simulink model "ee463_term_project"  (R2020a)
settings: Solver=VariableStepAuto  StartTime=0.0  StopTime=20  RelTol=1e-3
undefined symbols (not defined in the file): Acid, Lead
libraries: powerlib x25, electricdrivelib x1, powerlib_meascontrol x1, eePwmGenerator x1
settings Model: Creator=görkem  LastModifiedBy=görkem

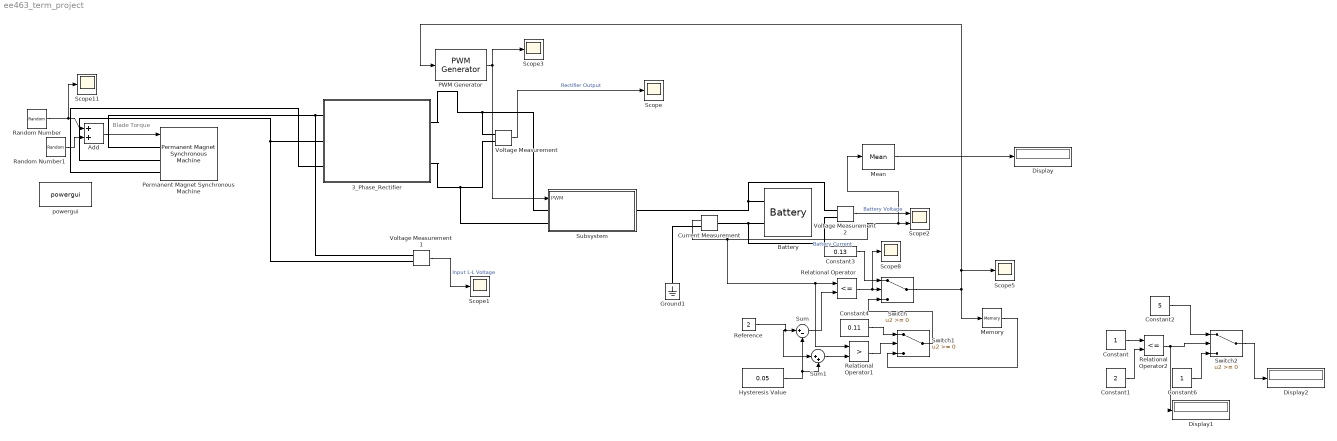
== system ee463_term_project ==
  note: Blade Torque
  3_Phase_Rectifier : Subsystem
  Add : Sum
  Battery : electricdrivelib/Extra Sources/Battery  BatType=Lead-Acid  ShowTempParam=off  ThermalPreset=no  ShowAgeParam=off  NomV=24  NomQ=5.4  SOC=50  Batt_Tr=30  PresetModel=on  MaxQ=5.625  MinV=18  FullV=26.1316  Dis_rate=1.08  R=0.044444  Normal_OP=1.6755  expZone="[24.4342        0.018]"  current=[6.5 13 32.5]  Units=Time  Tci=20  NomT=20  T2=-30  MaxQ2=4.8  FullV2=7.1  Normal_OP2=5.655  expZone2="[6.58           1]"  Rca=0.6  ti=2000  Dp=0  Neq0=0  Tsim=1e6  Ta1=25  Qeol=5.4*0.9  Reol=0.013333*1.2  Char_age=[2.3478, 3]  Dis_age=[2.3478, 10]  N1=1500  N2=10500  N3=1000  N4=1400  Ta2=45  N5=950
  Constant : Constant
  Constant1 : Constant  Value=2
  Constant2 : Constant  Value=5
  Constant3 : Constant  Value=0.13
  Constant4 : Constant  Value=0.11
  Constant6 : Constant
  Current Measurement : powerlib/Measurements/Current Measurement  PhasorSimulation=off  OutputType=Complex  PSBequivalent=0
  Display : Display
  Display1 : Display
  Display2 : Display
  Ground1 : powerlib/Elements/Ground  LConnTagsString=a
  Hysteresis Value : Constant  Value=0.05
  Mean : powerlib_meascontrol/Measurements/Mean  Freq=60  Vinit=0  Ts=0
  Memory : Memory
  PWM Generator : eePwmGenerator/PWM Generator  CarrCount=Up  Tper=0.0001  Ts=1e-5
  Permanent Magnet Synchronous Machine : powerlib/Machines/Permanent Magnet Synchronous Machine  NbPhases=3  FluxDistribution=Sinusoidal  RotorType=Round  MechanicalLoad=Torque Tm  PresetModel=No  ShowDetailedParameters=on  MeasurementBus=off  Resistance=10.58  Inductance=8.5e-3  dqInductances=[8.5e-3,8.5e-3]  La=0.0167  MachineConstant=Voltage Constant (V_peak L-L / krpm)  Flux=0.60646  VoltageCst=110  TorqueCst=0.90969  Flat=120  Mechanical=[0.00027 0.005024 1 0]  PolePairs=4  InitialConditions=[300,0, 0,0]  InitialConditions5ph=[0 0 0 0 0 0]  RefAngle=90 degrees behind phase A axis (modified Park)  IterativeDiscreteModel=Trapezoidal non iterative  TsBlock=-1  TsPowergui=0
  Random Number : RandomNumber  Mean=-1.6  Variance=0.05  SampleTime=1
  Random Number1 : RandomNumber  Variance=0.1  SampleTime=1e-3
  Reference : Constant  Value=2
  Relational Operator : RelationalOperator  Operator=<=  OutDataTypeStr=boolean  RndMeth=Simplest
  Relational Operator1 : RelationalOperator  Operator=>  OutDataTypeStr=boolean  RndMeth=Simplest
  Relational Operator2 : RelationalOperator  Operator=<=  OutDataTypeStr=boolean  RndMeth=Simplest
  Scope{,1,3,5,8,11} (6 alike) : Scope
  Scope2 : Scope  NumInputPorts=2
  Subsystem : Subsystem
  Sum : Sum  Inputs=|+-
  Sum1 : Sum  Inputs=|++
  Switch : Switch
  Switch1 : Switch
  Switch2 : Switch
  Voltage Measurement : powerlib/Measurements/Voltage Measurement  PhasorSimulation=off  OutputType=Complex  PSBequivalent=0
  Voltage Measurement1 : powerlib/Measurements/Voltage Measurement  PhasorSimulation=off  OutputType=Complex  PSBequivalent=0
  Voltage Measurement2 : powerlib/Measurements/Voltage Measurement  PhasorSimulation=off  OutputType=Complex  PSBequivalent=0
  powergui : powerlib/powergui  Priority=1  SimulationMode=Discrete  SampleTime=1e-5  frequency=60  Iterations=50  frequencyindice=0  Pbase=100e6  ErrMax=1e-4  UnitsV=kV  UnitsW=MW  buscounter=0  FunctionMessages=off  echomessages=off  EnableUseOfTLC=off  CurrentSourceSwitches=off  DisableSnubberDevices=off  DisableRonSwitches=off  DisableVfSwitches=off  DisplayEquations=off  AutomaticDiscreteSolvers=off  SolverType=Tustin/Backward Euler (TBE)  Interpol=off  ExternalGateDelay=off  methode=off  Ts=100  x0status=blocks  SPID=on  SwTol=0  HookPort=off  NonlinearTolerance=1e-4  nMaxIteration=100  ContinueOnMaxIteration=off  RestoreLinks=warning  ResistiveCurrentMeasurement=off  Frange=[0:2:500]  Ylog=off  Xlog=on  ShowGrid=off  save=off  variable=ZData  structure=0  ZoomFFT=off  StartTime=0.0  cycles=1  DisplayStyle=1  fundamental=60  FreqAxis=off  MaxFrequency=1000  frequencyindicesteady=1  RmsSteady=1  display=off
  wires:
  Voltage Measurement/1 -> Scope/1  "Rectifier Output"
  PWM Generator/1 -> Scope3/1, Subsystem/1(PWM)
  Random Number/1 -> Scope11/1, Add/1
  Add/1 -> Permanent Magnet Synchronous Machine/1
  Voltage Measurement1/1 -> Scope1/1  "Input L-L Voltage"
  Voltage Measurement2/1 -> Scope2/1  "Battery Voltage"
  Current Measurement/1 -> Relational Operator1/1, Relational Operator/1, Mean/1, Scope2/2  "Battery Current"
  Random Number1/1 -> Add/2
  Reference/1 -> Sum1/1, Sum/1
  Sum/1 -> Relational Operator/2
  Hysteresis Value/1 -> Sum/2, Sum1/2
  Sum1/1 -> Relational Operator1/2
  Constant3/1 -> Switch/1
  Relational Operator/1 -> Scope8/1, Switch/2
  Switch1/1 -> Switch/3
  Constant4/1 -> Switch1/1
  Relational Operator1/1 -> Switch1/2
  Memory/1 -> Switch1/3
  Mean/1 -> Display/1
  Constant/1 -> Relational Operator2/1
  Constant1/1 -> Relational Operator2/2
  Relational Operator2/1 -> Display1/1, Switch2/2
  Constant2/1 -> Switch2/1
  Constant6/1 -> Switch2/3
  Switch2/1 -> Display2/1
  Switch/1 -> PWM Generator/1, Scope5/1, Memory/1
  connections:
  Current Measurement/LConn1 -- Voltage Measurement2/LConn2 -- Battery/LConn2
  3_Phase_Rectifier/LConn1 -- Permanent Magnet Synchronous Machine/LConn1 -- Voltage Measurement1/LConn1
  3_Phase_Rectifier/RConn2 -- Voltage Measurement/LConn2 -- Subsystem/LConn2
  3_Phase_Rectifier/LConn2 -- Permanent Magnet Synchronous Machine/LConn2 -- Voltage Measurement1/LConn2
  Voltage Measurement/LConn1 -- 3_Phase_Rectifier/RConn1 -- Subsystem/LConn1
  Voltage Measurement2/LConn1 -- Subsystem/RConn1 -- Battery/LConn1
  Permanent Magnet Synchronous Machine/LConn3 -- 3_Phase_Rectifier/LConn3
  Ground1/LConn1 -- Current Measurement/RConn1

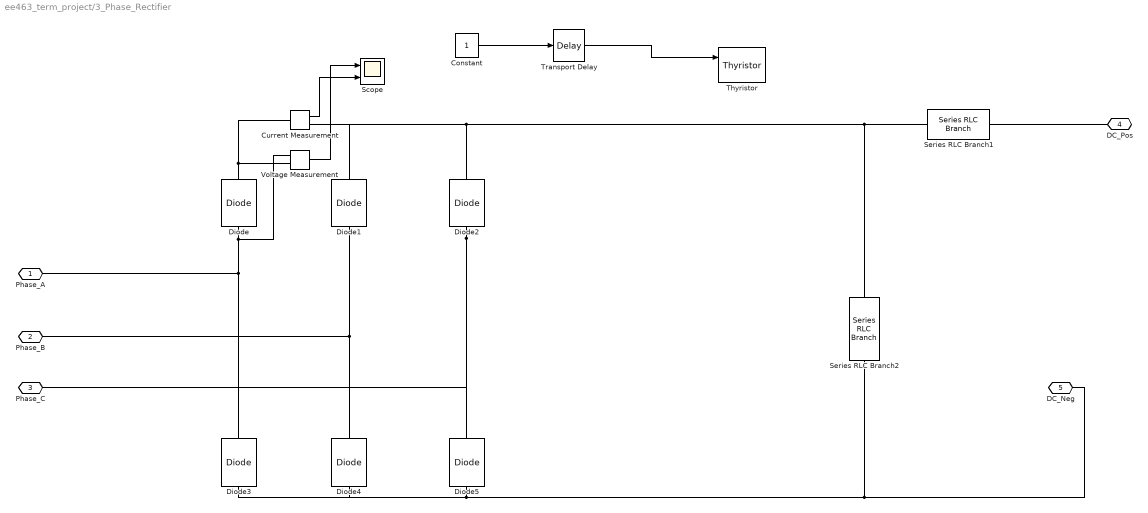
== system ee463_term_project/3_Phase_Rectifier ==
  Constant : Constant
  Current Measurement : powerlib/Measurements/Current Measurement  PhasorSimulation=off  OutputType=Complex  PSBequivalent=0
  Diode{,1..5} (6 alike) : powerlib/Power Electronics/Diode  Ron=0.001  Lon=0  Vf=0.8  IC=0  UseSnubber=0  Rs=500  Cs=250e-9  Measurements=off
  Scope : Scope  NumInputPorts=2
  Series RLC Branch1 : powerlib/Elements/Series RLC Branch  LConnTagsString=__new0  RConnTagsString=__new0  BranchType=R  Resistance=20  Inductance=1e-3  SetiL0=off  InitialCurrent=0  Capacitance=1e-6  Setx0=off  InitialVoltage=0  Measurements=None
  Series RLC Branch2 : powerlib/Elements/Series RLC Branch  LConnTagsString=__new0  RConnTagsString=__new0  BranchType=C  Resistance=72  Inductance=1e-3  SetiL0=off  InitialCurrent=0  Capacitance=1e-3  Setx0=off  InitialVoltage=0  Measurements=None
  Thyristor : powerlib/Power Electronics/Thyristor  Ron=0.001  Lon=0  Vf=0.8  IC=0  Rs=500  Cs=250e-9  Measurements=off
  Transport Delay : TransportDelay  DelayTime=0.2
  Voltage Measurement : powerlib/Measurements/Voltage Measurement  PhasorSimulation=off  OutputType=Complex  PSBequivalent=0
  Phase_A : PMIOPort  Side=Left
  Phase_B : PMIOPort  Port=2  Side=Left
  Phase_C : PMIOPort  Port=3  Side=Left
  DC_Pos : PMIOPort  Port=4  Side=Right
  DC_Neg : PMIOPort  Port=5  Side=Right
  wires:
  Transport Delay/1 -> Thyristor/1
  Constant/1 -> Transport Delay/1
  Voltage Measurement/1 -> Scope/1
  Current Measurement/1 -> Scope/2
  connections:
  Diode2/LConn1 -- Phase_C/RConn1 -- Diode5/RConn1
  Series RLC Branch2/LConn1 -- Current Measurement/RConn1 -- Diode1/RConn1 -- Diode2/RConn1 -- Series RLC Branch1/LConn1
  Series RLC Branch2/RConn1 -- Diode3/LConn1 -- Diode4/LConn1 -- Diode5/LConn1 -- DC_Neg/RConn1
  Phase_A/RConn1 -- Diode3/RConn1 -- Voltage Measurement/LConn1 -- Diode/LConn1
  Diode4/RConn1 -- Phase_B/RConn1 -- Diode1/LConn1
  Diode/RConn1 -- Current Measurement/LConn1 -- Voltage Measurement/LConn2
  Series RLC Branch1/RConn1 -- DC_Pos/RConn1

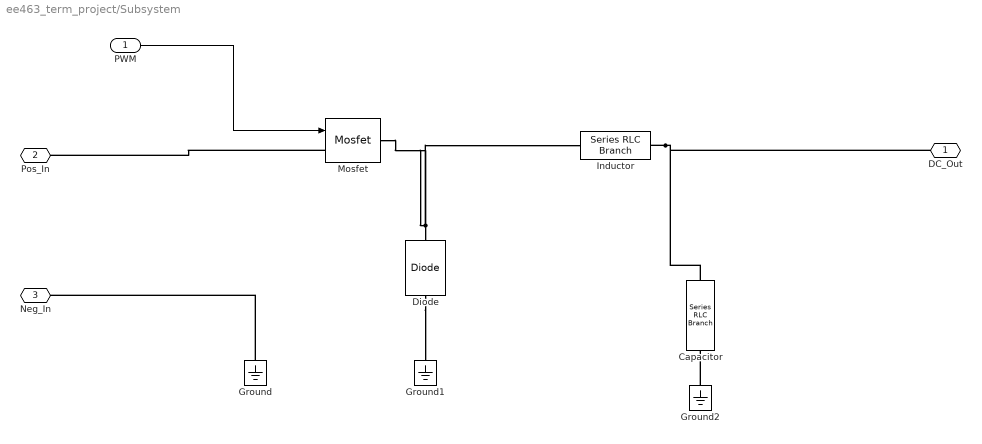
== system ee463_term_project/Subsystem ==
  PWM : Inport
  Capacitor : powerlib/Elements/Series RLC Branch  LConnTagsString=__new0  RConnTagsString=__new0  BranchType=C  Resistance=1  Inductance=1e-3  SetiL0=off  InitialCurrent=0  Capacitance=50e-6  Setx0=off  InitialVoltage=0  Measurements=None
  Diode : powerlib/Power Electronics/Diode  Ron=0.001  Lon=0  Vf=0.8  IC=0  UseSnubber=off  Rs=500  Cs=250e-9  Measurements=off
  Ground : powerlib/Elements/Ground  LConnTagsString=a
  Ground1 : powerlib/Elements/Ground  LConnTagsString=a
  Ground2 : powerlib/Elements/Ground  LConnTagsString=a
  Inductor : powerlib/Elements/Series RLC Branch  LConnTagsString=__new0  RConnTagsString=__new0  BranchType=L  Resistance=1  Inductance=5e-3  SetiL0=off  InitialCurrent=0  Capacitance=1e-6  Setx0=off  InitialVoltage=0  Measurements=None
  Mosfet : powerlib/Power Electronics/Mosfet  Ron=0.1  Lon=0  Rd=0.01  Vfd=0  IC=0  Rs=1e5  Cs=inf  Measurements=off
  DC_Out : PMIOPort  Side=Right
  Pos_In : PMIOPort  Port=2  Side=Left
  Neg_In : PMIOPort  Port=3  Side=Left
  wires:
  PWM/1 -> Mosfet/1
  connections:
  Ground2/LConn1 -- Capacitor/RConn1
  Diode/RConn1 -- Mosfet/RConn1 -- Inductor/LConn1
  Inductor/RConn1 -- Capacitor/LConn1 -- DC_Out/RConn1
  Diode/LConn1 -- Ground1/LConn1
  Mosfet/LConn1 -- Pos_In/RConn1
  Ground/LConn1 -- Neg_In/RConn1
